simulink model "chap9_4sim"  (Simulink 8.1)
settings: Solver=ode45  StartTime=0.0  StopTime=10.0  FixedStep=0.002  RelTol=1e-3
settings Model: Creator=liujk  LastModifiedBy=liujk
settings DataIOCC: SignalLoggingName=sigsOut
settings OptimizationCC: ExpressionDepthLimit=128
settings DebuggingCC: SaveWithParameterizedLinksMsg=none  SignalResolutionControl=TryResolveAllWithWarning  SolverPrmCheckMsg=none  MultiTaskDSMMsg=warning  MultiTaskCondExecSysMsg=none  StrictBusMsg=None
settings HardwareCC: TargetUnknown=on
settings RTWCC: IncludeERTFirstTime=on

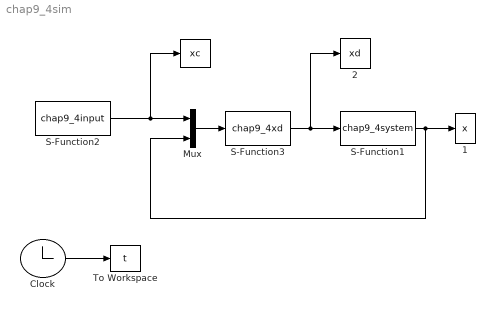
== system chap9_4sim ==
  "  " : ToWorkspace  VariableName=xc  SampleTime=-1
  "  1" : ToWorkspace  VariableName=x  SampleTime=-1
  "  2" : ToWorkspace  VariableName=xd  SampleTime=-1
  Clock : Clock
  Mux : Mux  Inputs=2
  S-Function1 : S-Function  FunctionName=chap9_4system  EnableBusSupport=off
  S-Function2 : S-Function  FunctionName=chap9_4input  EnableBusSupport=off
  S-Function3 : S-Function  FunctionName=chap9_4xd  EnableBusSupport=off
  To Workspace : ToWorkspace  VariableName=t  SampleTime=-1
  wires:
  S-Function1/1 -> "  1"/1, Mux/2
  Clock/1 -> To Workspace/1
  S-Function3/1 -> S-Function1/1, "  2"/1
  S-Function2/1 -> Mux/1, "  "/1
  Mux/1 -> S-Function3/1
